simulink model "gm_UZ_EnDat"  (R2023b)
settings: Solver=FixedStepDiscrete  StartTime=0  StopTime=0.002  RelTol=1e-3
model workspace (MAT data in the model file):
  Select = 0
libraries: hdlsllib x314, hdlmdlgenlib x10, simulink x7, simulink_extras x3
(part 6 of 7)

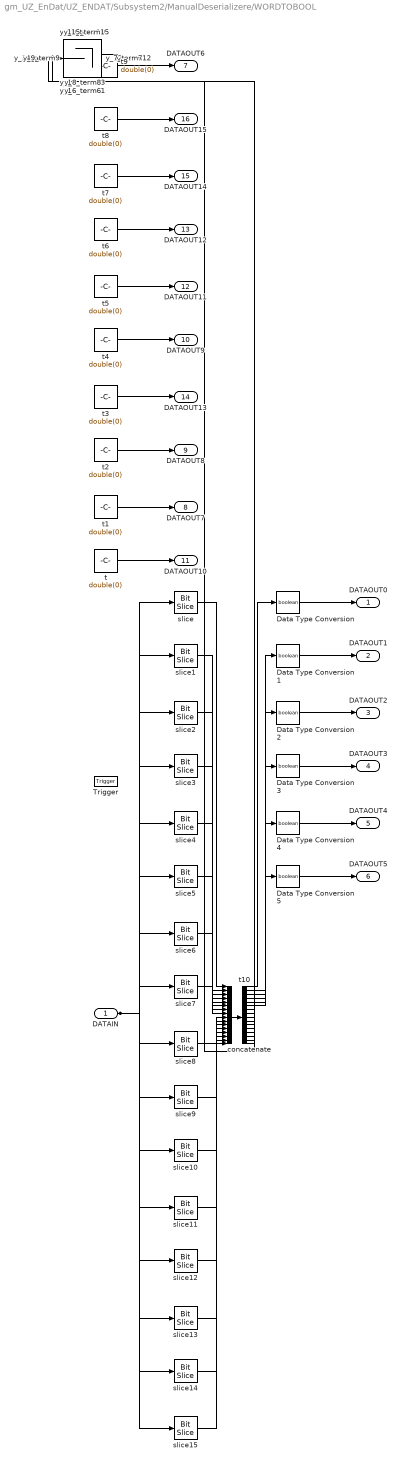
== system gm_UZ_EnDat/UZ_ENDAT/Subsystem2/ManualDeserializere/WORDTOBOOL ==
  DATAIN : Inport  OutDataTypeStr=uint16  PortDimensions=1
  Trigger : TriggerPort  TriggerType=falling  VariantControl=(inherit)  OutputDataType=int8  InitialTriggerSignalState=positive  PortDimensions=1  OutDataTypeStr=boolean
  Data Type Conversion{,1..5} (6 alike) : DataTypeConversion  OutDataTypeStr=boolean  SaturateOnIntegerOverflow=off  RndMeth=Floor
  concatenate : Concatenate  NumInputs=16  Mode=Multidimensional array  ConcatenateDimension=2
  slice : hdlsllib/Logic and Bit Operations/Bit Slice  lidx=double(0)  ridx=double(0)
  slice1 : hdlsllib/Logic and Bit Operations/Bit Slice  lidx=double(1)  ridx=double(1)
  slice10 : hdlsllib/Logic and Bit Operations/Bit Slice  lidx=double(10)  ridx=double(10)
  slice11 : hdlsllib/Logic and Bit Operations/Bit Slice  lidx=double(11)  ridx=double(11)
  slice12 : hdlsllib/Logic and Bit Operations/Bit Slice  lidx=double(12)  ridx=double(12)
  slice13 : hdlsllib/Logic and Bit Operations/Bit Slice  lidx=double(13)  ridx=double(13)
  slice14 : hdlsllib/Logic and Bit Operations/Bit Slice  lidx=double(14)  ridx=double(14)
  slice15 : hdlsllib/Logic and Bit Operations/Bit Slice  lidx=double(15)  ridx=double(15)
  slice2 : hdlsllib/Logic and Bit Operations/Bit Slice  lidx=double(2)  ridx=double(2)
  slice3 : hdlsllib/Logic and Bit Operations/Bit Slice  lidx=double(3)  ridx=double(3)
  slice4 : hdlsllib/Logic and Bit Operations/Bit Slice  lidx=double(4)  ridx=double(4)
  slice5 : hdlsllib/Logic and Bit Operations/Bit Slice  lidx=double(5)  ridx=double(5)
  slice6 : hdlsllib/Logic and Bit Operations/Bit Slice  lidx=double(6)  ridx=double(6)
  slice7 : hdlsllib/Logic and Bit Operations/Bit Slice  lidx=double(7)  ridx=double(7)
  slice8 : hdlsllib/Logic and Bit Operations/Bit Slice  lidx=double(8)  ridx=double(8)
  slice9 : hdlsllib/Logic and Bit Operations/Bit Slice  lidx=double(9)  ridx=double(9)
  t{,1..9} (10 alike) : Constant  Value=double(0)  OutDataTypeStr=boolean  SampleTime=-1
  t10 : Demux  Outputs=16
  y_10_term10 : Terminator
  y_11_term11 : Terminator
  y_12_term12 : Terminator
  y_13_term13 : Terminator
  y_14_term14 : Terminator
  y_15_term15 : Terminator
  y_6_term6 : Terminator
  y_7_term7 : Terminator
  y_8_term8 : Terminator
  y_9_term9 : Terminator
  DATAOUT0 : Outport  InitialOutput=0
  DATAOUT1 : Outport  Port=2  InitialOutput=0
  DATAOUT2 : Outport  Port=3  InitialOutput=0
  DATAOUT3 : Outport  Port=4  InitialOutput=0
  DATAOUT4 : Outport  Port=5  InitialOutput=0
  DATAOUT5 : Outport  Port=6  InitialOutput=0
  DATAOUT6 : Outport  Port=7  InitialOutput=0
  DATAOUT7 : Outport  Port=8  InitialOutput=0
  DATAOUT8 : Outport  Port=9  InitialOutput=0
  DATAOUT9 : Outport  Port=10  InitialOutput=0
  DATAOUT10 : Outport  Port=11  InitialOutput=0
  DATAOUT11 : Outport  Port=12  InitialOutput=0
  DATAOUT12 : Outport  Port=13  InitialOutput=0
  DATAOUT13 : Outport  Port=14  InitialOutput=0
  DATAOUT14 : Outport  Port=15  InitialOutput=0
  DATAOUT15 : Outport  Port=16  InitialOutput=0
  wires:
  DATAIN/1 -> slice15/1, slice14/1, slice13/1, slice12/1, slice11/1, slice10/1, slice9/1, slice8/1, slice7/1, slice6/1, slice5/1, slice4/1, slice3/1, slice2/1, slice1/1, slice/1
  Data Type Conversion/1 -> DATAOUT0/1
  Data Type Conversion1/1 -> DATAOUT1/1
  t/1 -> DATAOUT10/1
  t5/1 -> DATAOUT11/1
  t6/1 -> DATAOUT12/1
  t3/1 -> DATAOUT13/1
  t7/1 -> DATAOUT14/1
  t8/1 -> DATAOUT15/1
  Data Type Conversion2/1 -> DATAOUT2/1
  Data Type Conversion3/1 -> DATAOUT3/1
  Data Type Conversion4/1 -> DATAOUT4/1
  Data Type Conversion5/1 -> DATAOUT5/1
  t9/1 -> DATAOUT6/1
  t1/1 -> DATAOUT7/1
  t2/1 -> DATAOUT8/1
  t4/1 -> DATAOUT9/1
  concatenate/1 -> t10/1
  t10/1 -> Data Type Conversion/1
  t10/2 -> Data Type Conversion1/1
  t10/3 -> Data Type Conversion2/1
  t10/4 -> Data Type Conversion3/1
  t10/5 -> Data Type Conversion4/1
  t10/6 -> Data Type Conversion5/1
  t10/7 -> y_6_term6/1
  t10/8 -> y_7_term7/1
  t10/9 -> y_8_term8/1
  t10/10 -> y_9_term9/1
  t10/11 -> y_10_term10/1
  t10/12 -> y_11_term11/1
  t10/13 -> y_12_term12/1
  t10/14 -> y_13_term13/1
  t10/15 -> y_14_term14/1
  t10/16 -> y_15_term15/1
  slice/1 -> concatenate/1
  slice1/1 -> concatenate/2
  slice2/1 -> concatenate/3
  slice3/1 -> concatenate/4
  slice4/1 -> concatenate/5
  slice5/1 -> concatenate/6
  slice6/1 -> concatenate/7
  slice7/1 -> concatenate/8
  slice8/1 -> concatenate/9
  slice9/1 -> concatenate/10
  slice10/1 -> concatenate/11
  slice11/1 -> concatenate/12
  slice12/1 -> concatenate/13
  slice13/1 -> concatenate/14
  slice14/1 -> concatenate/15
  slice15/1 -> concatenate/16

== system gm_UZ_EnDat/UZ_ENDAT/Subsystem2/ManualDeserializere/ramwatcher ==
  In1 : Inport  OutMin=0  OutMax=32000  OutDataTypeStr=uint16  PortDimensions=1  LockScale=on
  reset : Inport  Port=2  OutMin=0  OutMax=1  OutDataTypeStr=boolean  PortDimensions=1  LockScale=on
  Trigger : TriggerPort  VariantControl=(inherit)  OutputDataType=int8  InitialTriggerSignalState=zero  PortDimensions=1  OutDataTypeStr=boolean
  Constant2 : Constant  Value=0  OutDataTypeStr=uint16  SampleTime=-1
  Increment Stored Integer : Subsystem  mask(Stored Integer Value Increment){}
      mask help: Simulink:masks:StoredIntegerValueIncrement_MD
      mask Display: disp('Q++')
  Index Vector1 : MultiPortSwitch  DataPortOrder=Zero-based contiguous  Inputs=2  DiagnosticForDefault=None  zeroidx=on  OutDataTypeStr=uint16  SaturateOnIntegerOverflow=off  InputSameDT=off
  SEL : Outport  InitialOutput=0
  wires:
  In1/1 -> Increment Stored Integer/1(u)
  reset/1 -> Index Vector1/1
  Constant2/1 -> Index Vector1/3
  Increment Stored Integer/1(y) -> Index Vector1/2
  Index Vector1/1 -> SEL/1

== system gm_UZ_EnDat/UZ_ENDAT/timingprovider/CLKCNTER_POSCNTR/Positional_Counter ==
  valueout : Inport  OutDataTypeStr=uint32  PortDimensions=1
  Trigger : TriggerPort  VariantControl=(inherit)  InitialTriggerSignalState=zero  PortDimensions=1  OutDataTypeStr=boolean
  Increment Stored Integer : Subsystem  mask(Stored Integer Value Increment){}
      mask help: Simulink:masks:StoredIntegerValueIncrement_MD
      mask Display: disp('Q++')
  divider : Outport  InitialOutput=0
  wires:
  valueout/1 -> Increment Stored Integer/1(u)
  Increment Stored Integer/1(y) -> divider/1

== system gm_UZ_EnDat/UZ_ENDAT/timingprovider/CLKCNTER_POSCNTR/SetZero32modified ==
  valin : Inport  OutDataTypeStr=uint32  PortDimensions=1
  setzero : Inport  Port=2  OutDataTypeStr=boolean  PortDimensions=1
  Trigger : TriggerPort  TriggerType=either  VariantControl=(inherit)  PortDimensions=1  OutDataTypeStr=boolean
  Constant2 : Constant  Value=0  OutDataTypeStr=uint32  SampleTime=-1
  Index Vector1 : MultiPortSwitch  DataPortOrder=Zero-based contiguous  Inputs=2  DiagnosticForDefault=None  zeroidx=on  OutDataTypeStr=uint32  SaturateOnIntegerOverflow=off  InputSameDT=off
  valueout : Outport  InitialOutput=0  VectorParamsAs1DForOutWhenUnconnected=off
  wires:
  valin/1 -> Index Vector1/2
  setzero/1 -> Index Vector1/1
  Constant2/1 -> Index Vector1/3
  Index Vector1/1 -> valueout/1

== system gm_UZ_EnDat/UZ_ENDAT/timingprovider/CLKCNTER_POSCNTR/SetZero32modified1 ==
  valin : Inport  OutDataTypeStr=uint32  PortDimensions=1
  setzero : Inport  Port=2  OutDataTypeStr=boolean  PortDimensions=1
  Trigger : TriggerPort  TriggerType=either  VariantControl=(inherit)  PortDimensions=1  OutDataTypeStr=boolean
  Constant2 : Constant  Value=0  OutDataTypeStr=uint32  SampleTime=-1
  Index Vector1 : MultiPortSwitch  DataPortOrder=Zero-based contiguous  Inputs=2  DiagnosticForDefault=None  zeroidx=on  OutDataTypeStr=uint32  SaturateOnIntegerOverflow=off  InputSameDT=off
  valueout : Outport  InitialOutput=0  VectorParamsAs1DForOutWhenUnconnected=off
  wires:
  valin/1 -> Index Vector1/2
  setzero/1 -> Index Vector1/1
  Constant2/1 -> Index Vector1/3
  Index Vector1/1 -> valueout/1

== system gm_UZ_EnDat/UZ_ENDAT/timingprovider/CLKCNTER_POSCNTR1/Positional_Counter ==
  valueout : Inport  OutDataTypeStr=uint32  PortDimensions=1
  Trigger : TriggerPort  VariantControl=(inherit)  InitialTriggerSignalState=zero  PortDimensions=1  OutDataTypeStr=boolean
  Increment Stored Integer : Subsystem  mask(Stored Integer Value Increment){}
      mask help: Simulink:masks:StoredIntegerValueIncrement_MD
      mask Display: disp('Q++')
  divider : Outport  InitialOutput=0
  wires:
  Increment Stored Integer/1(y) -> divider/1
  valueout/1 -> Increment Stored Integer/1(u)

== system gm_UZ_EnDat/UZ_ENDAT/timingprovider/CLKCNTER_POSCNTR1/SetZero32modified ==
  valin : Inport  OutDataTypeStr=uint32  PortDimensions=1
  setzero : Inport  Port=2  OutDataTypeStr=boolean  PortDimensions=1
  Trigger : TriggerPort  TriggerType=either  VariantControl=(inherit)  PortDimensions=1  OutDataTypeStr=boolean
  Constant2 : Constant  Value=0  OutDataTypeStr=uint32  SampleTime=-1
  Index Vector1 : MultiPortSwitch  DataPortOrder=Zero-based contiguous  Inputs=2  DiagnosticForDefault=None  zeroidx=on  OutDataTypeStr=uint32  SaturateOnIntegerOverflow=off  InputSameDT=off
  valueout : Outport  InitialOutput=0  VectorParamsAs1DForOutWhenUnconnected=off
  wires:
  Constant2/1 -> Index Vector1/3
  Index Vector1/1 -> valueout/1
  valin/1 -> Index Vector1/2
  setzero/1 -> Index Vector1/1

== system gm_UZ_EnDat/UZ_ENDAT/timingprovider/Subsystem2/Compare To Constant1 ==
  u : Inport  OutDataTypeStr=uint32  SampleTime=1e-08
  Compare : RelationalOperator  Operator===  OutDataTypeStr=boolean
  Constant : Constant  DisableCoverage=on  Value=const  OutDataTypeStr=Inherit: Inherit via back propagation  SampleTime=-1
  y : Outport  SampleTime=1e-08
  wires:
  u/1 -> Compare/1
  Compare/1 -> y/1
  Constant/1 -> Compare/2

== system gm_UZ_EnDat/UZ_ENDAT/timingprovider/Subsystem2/Detect Increase ==
  note: U(k)
  note: Edge
  U : Inport  OutDataTypeStr=boolean  SampleTime=1e-08
  Delay Input1 : UnitDelay  SampleTime=1e-08
  FixPt Relational Operator : RelationalOperator  Operator=>  OutDataTypeStr=boolean  SampleTime=1e-08  InputSameDT=off
  Y : Outport  SampleTime=1e-08
  wires:
  U/1 -> FixPt Relational Operator/1, Delay Input1/1
  Delay Input1/1 -> FixPt Relational Operator/2
  FixPt Relational Operator/1 -> Y/1

== system gm_UZ_EnDat/UZ_ENDAT/timingprovider/Subsystem3/Compare To Constant1 ==
  u : Inport  OutDataTypeStr=uint32  SampleTime=1e-08
  Compare : RelationalOperator  Operator===  OutDataTypeStr=boolean
  Constant : Constant  DisableCoverage=on  Value=const  OutDataTypeStr=Inherit: Inherit via back propagation  SampleTime=-1
  y : Outport  SampleTime=1e-08
  wires:
  u/1 -> Compare/1
  Compare/1 -> y/1
  Constant/1 -> Compare/2

== system gm_UZ_EnDat/UZ_ENDAT/timingprovider/Subsystem3/Detect Increase ==
  note: U(k)
  note: Edge
  U : Inport  OutDataTypeStr=boolean  SampleTime=1e-08
  Delay Input1 : UnitDelay  SampleTime=1e-08
  FixPt Relational Operator : RelationalOperator  Operator=>  OutDataTypeStr=boolean  SampleTime=1e-08  InputSameDT=off
  Y : Outport  SampleTime=1e-08
  wires:
  U/1 -> FixPt Relational Operator/1, Delay Input1/1
  Delay Input1/1 -> FixPt Relational Operator/2
  FixPt Relational Operator/1 -> Y/1

== system gm_UZ_EnDat/UZ_ENDAT/3timestorage/Triggered Subsystem/Counter Limited/Increment Real World ==
  u : Inport  OutDataTypeStr=uint8
  FixPt Constant : Constant  OutDataTypeStr=uint8  SampleTime=-1
  FixPt Data Type Duplicate : DataTypeDuplicate  DisableCoverage=on  NumInputPorts=3
  FixPt Sum1 : Sum  OutDataTypeStr=uint8  AccumDataTypeStr=uint8
  y : Outport  InitialOutput=0
  wires:
  u/1 -> FixPt Sum1/1, FixPt Data Type Duplicate/2
  FixPt Constant/1 -> FixPt Sum1/2, FixPt Data Type Duplicate/3
  FixPt Sum1/1 -> FixPt Data Type Duplicate/1, y/1

== system gm_UZ_EnDat/UZ_ENDAT/3timestorage/Triggered Subsystem/Counter Limited/Wrap To Zero ==
  note: U(k)
  U : Inport  OutDataTypeStr=uint8
  Constant : Constant  Value=0  OutDataTypeStr=uint8  SampleTime=-1
  FixPt Data Type Duplicate1 : DataTypeDuplicate  DisableCoverage=on  NumInputPorts=3
  FixPt Switch : Switch  Criteria=u2 > Threshold  Threshold=double(2)  OutDataTypeStr=uint8  SaturateOnIntegerOverflow=off  InputSameDT=off
  Y : Outport  InitialOutput=0
  wires:
  U/1 -> FixPt Switch/3, FixPt Switch/2, FixPt Data Type Duplicate1/2
  Constant/1 -> FixPt Switch/1, FixPt Data Type Duplicate1/3
  FixPt Switch/1 -> FixPt Data Type Duplicate1/1, Y/1

== system gm_UZ_EnDat/UZ_ENDAT/ManualSerialize/padder/nibblepadding1/padding1 ==
  in : Inport  OutDataTypeStr=fixdt(0, 64, 0)  PortDimensions=1  SampleTime=1e-08
  Bit Shift2 : hdlsllib/Logic and Bit Operations/Bit Shift  mode=Shift Right Logical  N=double(1)
  Bit Slice2 : hdlsllib/Logic and Bit Operations/Bit Slice  lidx=double(0)  ridx=double(0)
  Data Type Conversion2 : DataTypeConversion  OutDataTypeStr=boolean  RndMeth=Nearest  SampleTime=1e-08  SaturateOnIntegerOverflow=off
  Switch2 : Switch  Criteria=u2 > Threshold  Threshold=double(0)  OutDataTypeStr=fixdt(0, 64, 0)  SampleTime=1e-08  SaturateOnIntegerOverflow=off  InputSameDT=off
  out : Outport  SampleTime=1e-08
  wires:
  in/1 -> Switch2/1, Bit Slice2/1, Bit Shift2/1
  Bit Shift2/1 -> Switch2/3
  Bit Slice2/1 -> Data Type Conversion2/1
  Data Type Conversion2/1 -> Switch2/2
  Switch2/1 -> out/1

== system gm_UZ_EnDat/UZ_ENDAT/ManualSerialize/padder/nibblepadding1/padding2 ==
  in : Inport  OutDataTypeStr=fixdt(0, 64, 0)  PortDimensions=1  SampleTime=1e-08
  Bit Shift2 : hdlsllib/Logic and Bit Operations/Bit Shift  mode=Shift Right Logical  N=double(1)
  Bit Slice2 : hdlsllib/Logic and Bit Operations/Bit Slice  lidx=double(0)  ridx=double(0)
  Data Type Conversion2 : DataTypeConversion  OutDataTypeStr=boolean  RndMeth=Nearest  SampleTime=1e-08  SaturateOnIntegerOverflow=off
  Switch2 : Switch  Criteria=u2 > Threshold  Threshold=double(0)  OutDataTypeStr=fixdt(0, 64, 0)  SampleTime=1e-08  SaturateOnIntegerOverflow=off  InputSameDT=off
  out : Outport  SampleTime=1e-08
  wires:
  Switch2/1 -> out/1
  Data Type Conversion2/1 -> Switch2/2
  Bit Slice2/1 -> Data Type Conversion2/1
  Bit Shift2/1 -> Switch2/3
  in/1 -> Bit Shift2/1, Bit Slice2/1, Switch2/1

== system gm_UZ_EnDat/UZ_ENDAT/ManualSerialize/padder/nibblepadding1/padding3 ==
  in : Inport  OutDataTypeStr=fixdt(0, 64, 0)  PortDimensions=1  SampleTime=1e-08
  Bit Shift2 : hdlsllib/Logic and Bit Operations/Bit Shift  mode=Shift Right Logical  N=double(1)
  Bit Slice2 : hdlsllib/Logic and Bit Operations/Bit Slice  lidx=double(0)  ridx=double(0)
  Data Type Conversion2 : DataTypeConversion  OutDataTypeStr=boolean  RndMeth=Nearest  SampleTime=1e-08  SaturateOnIntegerOverflow=off
  Switch2 : Switch  Criteria=u2 > Threshold  Threshold=double(0)  OutDataTypeStr=fixdt(0, 64, 0)  SampleTime=1e-08  SaturateOnIntegerOverflow=off  InputSameDT=off
  out : Outport  SampleTime=1e-08
  wires:
  Switch2/1 -> out/1
  Data Type Conversion2/1 -> Switch2/2
  Bit Slice2/1 -> Data Type Conversion2/1
  Bit Shift2/1 -> Switch2/3
  in/1 -> Bit Shift2/1, Bit Slice2/1, Switch2/1

== system gm_UZ_EnDat/UZ_ENDAT/ManualSerialize/padder/nibblepadding10/padding1 ==
  in : Inport  OutDataTypeStr=fixdt(0, 64, 0)  PortDimensions=1  SampleTime=1e-08
  Bit Shift2 : hdlsllib/Logic and Bit Operations/Bit Shift  mode=Shift Right Logical  N=double(1)
  Bit Slice2 : hdlsllib/Logic and Bit Operations/Bit Slice  lidx=double(0)  ridx=double(0)
  Data Type Conversion2 : DataTypeConversion  OutDataTypeStr=boolean  RndMeth=Nearest  SampleTime=1e-08  SaturateOnIntegerOverflow=off
  Switch2 : Switch  Criteria=u2 > Threshold  Threshold=double(0)  OutDataTypeStr=fixdt(0, 64, 0)  SampleTime=1e-08  SaturateOnIntegerOverflow=off  InputSameDT=off
  out : Outport  SampleTime=1e-08
  wires:
  Switch2/1 -> out/1
  Data Type Conversion2/1 -> Switch2/2
  Bit Slice2/1 -> Data Type Conversion2/1
  Bit Shift2/1 -> Switch2/3
  in/1 -> Bit Shift2/1, Bit Slice2/1, Switch2/1

== system gm_UZ_EnDat/UZ_ENDAT/ManualSerialize/padder/nibblepadding10/padding2 ==
  in : Inport  OutDataTypeStr=fixdt(0, 64, 0)  PortDimensions=1  SampleTime=1e-08
  Bit Shift2 : hdlsllib/Logic and Bit Operations/Bit Shift  mode=Shift Right Logical  N=double(1)
  Bit Slice2 : hdlsllib/Logic and Bit Operations/Bit Slice  lidx=double(0)  ridx=double(0)
  Data Type Conversion2 : DataTypeConversion  OutDataTypeStr=boolean  RndMeth=Nearest  SampleTime=1e-08  SaturateOnIntegerOverflow=off
  Switch2 : Switch  Criteria=u2 > Threshold  Threshold=double(0)  OutDataTypeStr=fixdt(0, 64, 0)  SampleTime=1e-08  SaturateOnIntegerOverflow=off  InputSameDT=off
  out : Outport  SampleTime=1e-08
  wires:
  in/1 -> Switch2/1, Bit Slice2/1, Bit Shift2/1
  Bit Shift2/1 -> Switch2/3
  Bit Slice2/1 -> Data Type Conversion2/1
  Data Type Conversion2/1 -> Switch2/2
  Switch2/1 -> out/1

== system gm_UZ_EnDat/UZ_ENDAT/ManualSerialize/padder/nibblepadding10/padding3 ==
  in : Inport  OutDataTypeStr=fixdt(0, 64, 0)  PortDimensions=1  SampleTime=1e-08
  Bit Shift2 : hdlsllib/Logic and Bit Operations/Bit Shift  mode=Shift Right Logical  N=double(1)
  Bit Slice2 : hdlsllib/Logic and Bit Operations/Bit Slice  lidx=double(0)  ridx=double(0)
  Data Type Conversion2 : DataTypeConversion  OutDataTypeStr=boolean  RndMeth=Nearest  SampleTime=1e-08  SaturateOnIntegerOverflow=off
  Switch2 : Switch  Criteria=u2 > Threshold  Threshold=double(0)  OutDataTypeStr=fixdt(0, 64, 0)  SampleTime=1e-08  SaturateOnIntegerOverflow=off  InputSameDT=off
  out : Outport  SampleTime=1e-08
  wires:
  in/1 -> Switch2/1, Bit Slice2/1, Bit Shift2/1
  Bit Shift2/1 -> Switch2/3
  Bit Slice2/1 -> Data Type Conversion2/1
  Data Type Conversion2/1 -> Switch2/2
  Switch2/1 -> out/1

== system gm_UZ_EnDat/UZ_ENDAT/ManualSerialize/padder/nibblepadding11/padding1 ==
  in : Inport  OutDataTypeStr=fixdt(0, 64, 0)  PortDimensions=1  SampleTime=1e-08
  Bit Shift2 : hdlsllib/Logic and Bit Operations/Bit Shift  mode=Shift Right Logical  N=double(1)
  Bit Slice2 : hdlsllib/Logic and Bit Operations/Bit Slice  lidx=double(0)  ridx=double(0)
  Data Type Conversion2 : DataTypeConversion  OutDataTypeStr=boolean  RndMeth=Nearest  SampleTime=1e-08  SaturateOnIntegerOverflow=off
  Switch2 : Switch  Criteria=u2 > Threshold  Threshold=double(0)  OutDataTypeStr=fixdt(0, 64, 0)  SampleTime=1e-08  SaturateOnIntegerOverflow=off  InputSameDT=off
  out : Outport  SampleTime=1e-08
  wires:
  Switch2/1 -> out/1
  Data Type Conversion2/1 -> Switch2/2
  Bit Slice2/1 -> Data Type Conversion2/1
  Bit Shift2/1 -> Switch2/3
  in/1 -> Bit Shift2/1, Bit Slice2/1, Switch2/1

== system gm_UZ_EnDat/UZ_ENDAT/ManualSerialize/padder/nibblepadding11/padding2 ==
  in : Inport  OutDataTypeStr=fixdt(0, 64, 0)  PortDimensions=1  SampleTime=1e-08
  Bit Shift2 : hdlsllib/Logic and Bit Operations/Bit Shift  mode=Shift Right Logical  N=double(1)
  Bit Slice2 : hdlsllib/Logic and Bit Operations/Bit Slice  lidx=double(0)  ridx=double(0)
  Data Type Conversion2 : DataTypeConversion  OutDataTypeStr=boolean  RndMeth=Nearest  SampleTime=1e-08  SaturateOnIntegerOverflow=off
  Switch2 : Switch  Criteria=u2 > Threshold  Threshold=double(0)  OutDataTypeStr=fixdt(0, 64, 0)  SampleTime=1e-08  SaturateOnIntegerOverflow=off  InputSameDT=off
  out : Outport  SampleTime=1e-08
  wires:
  in/1 -> Switch2/1, Bit Slice2/1, Bit Shift2/1
  Bit Shift2/1 -> Switch2/3
  Bit Slice2/1 -> Data Type Conversion2/1
  Data Type Conversion2/1 -> Switch2/2
  Switch2/1 -> out/1

== system gm_UZ_EnDat/UZ_ENDAT/ManualSerialize/padder/nibblepadding11/padding3 ==
  in : Inport  OutDataTypeStr=fixdt(0, 64, 0)  PortDimensions=1  SampleTime=1e-08
  Bit Shift2 : hdlsllib/Logic and Bit Operations/Bit Shift  mode=Shift Right Logical  N=double(1)
  Bit Slice2 : hdlsllib/Logic and Bit Operations/Bit Slice  lidx=double(0)  ridx=double(0)
  Data Type Conversion2 : DataTypeConversion  OutDataTypeStr=boolean  RndMeth=Nearest  SampleTime=1e-08  SaturateOnIntegerOverflow=off
  Switch2 : Switch  Criteria=u2 > Threshold  Threshold=double(0)  OutDataTypeStr=fixdt(0, 64, 0)  SampleTime=1e-08  SaturateOnIntegerOverflow=off  InputSameDT=off
  out : Outport  SampleTime=1e-08
  wires:
  in/1 -> Switch2/1, Bit Slice2/1, Bit Shift2/1
  Bit Shift2/1 -> Switch2/3
  Bit Slice2/1 -> Data Type Conversion2/1
  Data Type Conversion2/1 -> Switch2/2
  Switch2/1 -> out/1

== system gm_UZ_EnDat/UZ_ENDAT/ManualSerialize/padder/nibblepadding12/padding1 ==
  in : Inport  OutDataTypeStr=fixdt(0, 64, 0)  PortDimensions=1  SampleTime=1e-08
  Bit Shift2 : hdlsllib/Logic and Bit Operations/Bit Shift  mode=Shift Right Logical  N=double(1)
  Bit Slice2 : hdlsllib/Logic and Bit Operations/Bit Slice  lidx=double(0)  ridx=double(0)
  Data Type Conversion2 : DataTypeConversion  OutDataTypeStr=boolean  RndMeth=Nearest  SampleTime=1e-08  SaturateOnIntegerOverflow=off
  Switch2 : Switch  Criteria=u2 > Threshold  Threshold=double(0)  OutDataTypeStr=fixdt(0, 64, 0)  SampleTime=1e-08  SaturateOnIntegerOverflow=off  InputSameDT=off
  out : Outport  SampleTime=1e-08
  wires:
  Switch2/1 -> out/1
  Data Type Conversion2/1 -> Switch2/2
  Bit Slice2/1 -> Data Type Conversion2/1
  Bit Shift2/1 -> Switch2/3
  in/1 -> Bit Shift2/1, Bit Slice2/1, Switch2/1

== system gm_UZ_EnDat/UZ_ENDAT/ManualSerialize/padder/nibblepadding12/padding2 ==
  in : Inport  OutDataTypeStr=fixdt(0, 64, 0)  PortDimensions=1  SampleTime=1e-08
  Bit Shift2 : hdlsllib/Logic and Bit Operations/Bit Shift  mode=Shift Right Logical  N=double(1)
  Bit Slice2 : hdlsllib/Logic and Bit Operations/Bit Slice  lidx=double(0)  ridx=double(0)
  Data Type Conversion2 : DataTypeConversion  OutDataTypeStr=boolean  RndMeth=Nearest  SampleTime=1e-08  SaturateOnIntegerOverflow=off
  Switch2 : Switch  Criteria=u2 > Threshold  Threshold=double(0)  OutDataTypeStr=fixdt(0, 64, 0)  SampleTime=1e-08  SaturateOnIntegerOverflow=off  InputSameDT=off
  out : Outport  SampleTime=1e-08
  wires:
  in/1 -> Switch2/1, Bit Slice2/1, Bit Shift2/1
  Bit Shift2/1 -> Switch2/3
  Bit Slice2/1 -> Data Type Conversion2/1
  Data Type Conversion2/1 -> Switch2/2
  Switch2/1 -> out/1

== system gm_UZ_EnDat/UZ_ENDAT/ManualSerialize/padder/nibblepadding12/padding3 ==
  in : Inport  OutDataTypeStr=fixdt(0, 64, 0)  PortDimensions=1  SampleTime=1e-08
  Bit Shift2 : hdlsllib/Logic and Bit Operations/Bit Shift  mode=Shift Right Logical  N=double(1)
  Bit Slice2 : hdlsllib/Logic and Bit Operations/Bit Slice  lidx=double(0)  ridx=double(0)
  Data Type Conversion2 : DataTypeConversion  OutDataTypeStr=boolean  RndMeth=Nearest  SampleTime=1e-08  SaturateOnIntegerOverflow=off
  Switch2 : Switch  Criteria=u2 > Threshold  Threshold=double(0)  OutDataTypeStr=fixdt(0, 64, 0)  SampleTime=1e-08  SaturateOnIntegerOverflow=off  InputSameDT=off
  out : Outport  SampleTime=1e-08
  wires:
  in/1 -> Switch2/1, Bit Slice2/1, Bit Shift2/1
  Bit Shift2/1 -> Switch2/3
  Bit Slice2/1 -> Data Type Conversion2/1
  Data Type Conversion2/1 -> Switch2/2
  Switch2/1 -> out/1

== system gm_UZ_EnDat/UZ_ENDAT/ManualSerialize/padder/nibblepadding13/padding1 ==
  in : Inport  OutDataTypeStr=fixdt(0, 64, 0)  PortDimensions=1  SampleTime=1e-08
  Bit Shift2 : hdlsllib/Logic and Bit Operations/Bit Shift  mode=Shift Right Logical  N=double(1)
  Bit Slice2 : hdlsllib/Logic and Bit Operations/Bit Slice  lidx=double(0)  ridx=double(0)
  Data Type Conversion2 : DataTypeConversion  OutDataTypeStr=boolean  RndMeth=Nearest  SampleTime=1e-08  SaturateOnIntegerOverflow=off
  Switch2 : Switch  Criteria=u2 > Threshold  Threshold=double(0)  OutDataTypeStr=fixdt(0, 64, 0)  SampleTime=1e-08  SaturateOnIntegerOverflow=off  InputSameDT=off
  out : Outport  SampleTime=1e-08
  wires:
  Switch2/1 -> out/1
  Data Type Conversion2/1 -> Switch2/2
  Bit Slice2/1 -> Data Type Conversion2/1
  Bit Shift2/1 -> Switch2/3
  in/1 -> Bit Shift2/1, Bit Slice2/1, Switch2/1

== system gm_UZ_EnDat/UZ_ENDAT/ManualSerialize/padder/nibblepadding13/padding2 ==
  in : Inport  OutDataTypeStr=fixdt(0, 64, 0)  PortDimensions=1  SampleTime=1e-08
  Bit Shift2 : hdlsllib/Logic and Bit Operations/Bit Shift  mode=Shift Right Logical  N=double(1)
  Bit Slice2 : hdlsllib/Logic and Bit Operations/Bit Slice  lidx=double(0)  ridx=double(0)
  Data Type Conversion2 : DataTypeConversion  OutDataTypeStr=boolean  RndMeth=Nearest  SampleTime=1e-08  SaturateOnIntegerOverflow=off
  Switch2 : Switch  Criteria=u2 > Threshold  Threshold=double(0)  OutDataTypeStr=fixdt(0, 64, 0)  SampleTime=1e-08  SaturateOnIntegerOverflow=off  InputSameDT=off
  out : Outport  SampleTime=1e-08
  wires:
  in/1 -> Switch2/1, Bit Slice2/1, Bit Shift2/1
  Bit Shift2/1 -> Switch2/3
  Bit Slice2/1 -> Data Type Conversion2/1
  Data Type Conversion2/1 -> Switch2/2
  Switch2/1 -> out/1

== system gm_UZ_EnDat/UZ_ENDAT/ManualSerialize/padder/nibblepadding13/padding3 ==
  in : Inport  OutDataTypeStr=fixdt(0, 64, 0)  PortDimensions=1  SampleTime=1e-08
  Bit Shift2 : hdlsllib/Logic and Bit Operations/Bit Shift  mode=Shift Right Logical  N=double(1)
  Bit Slice2 : hdlsllib/Logic and Bit Operations/Bit Slice  lidx=double(0)  ridx=double(0)
  Data Type Conversion2 : DataTypeConversion  OutDataTypeStr=boolean  RndMeth=Nearest  SampleTime=1e-08  SaturateOnIntegerOverflow=off
  Switch2 : Switch  Criteria=u2 > Threshold  Threshold=double(0)  OutDataTypeStr=fixdt(0, 64, 0)  SampleTime=1e-08  SaturateOnIntegerOverflow=off  InputSameDT=off
  out : Outport  SampleTime=1e-08
  wires:
  in/1 -> Switch2/1, Bit Slice2/1, Bit Shift2/1
  Bit Shift2/1 -> Switch2/3
  Bit Slice2/1 -> Data Type Conversion2/1
  Data Type Conversion2/1 -> Switch2/2
  Switch2/1 -> out/1

== system gm_UZ_EnDat/UZ_ENDAT/ManualSerialize/padder/nibblepadding14/padding1 ==
  in : Inport  OutDataTypeStr=fixdt(0, 64, 0)  PortDimensions=1  SampleTime=1e-08
  Bit Shift2 : hdlsllib/Logic and Bit Operations/Bit Shift  mode=Shift Right Logical  N=double(1)
  Bit Slice2 : hdlsllib/Logic and Bit Operations/Bit Slice  lidx=double(0)  ridx=double(0)
  Data Type Conversion2 : DataTypeConversion  OutDataTypeStr=boolean  RndMeth=Nearest  SampleTime=1e-08  SaturateOnIntegerOverflow=off
  Switch2 : Switch  Criteria=u2 > Threshold  Threshold=double(0)  OutDataTypeStr=fixdt(0, 64, 0)  SampleTime=1e-08  SaturateOnIntegerOverflow=off  InputSameDT=off
  out : Outport  SampleTime=1e-08
  wires:
  Switch2/1 -> out/1
  Data Type Conversion2/1 -> Switch2/2
  Bit Slice2/1 -> Data Type Conversion2/1
  Bit Shift2/1 -> Switch2/3
  in/1 -> Bit Shift2/1, Bit Slice2/1, Switch2/1

== system gm_UZ_EnDat/UZ_ENDAT/ManualSerialize/padder/nibblepadding14/padding2 ==
  in : Inport  OutDataTypeStr=fixdt(0, 64, 0)  PortDimensions=1  SampleTime=1e-08
  Bit Shift2 : hdlsllib/Logic and Bit Operations/Bit Shift  mode=Shift Right Logical  N=double(1)
  Bit Slice2 : hdlsllib/Logic and Bit Operations/Bit Slice  lidx=double(0)  ridx=double(0)
  Data Type Conversion2 : DataTypeConversion  OutDataTypeStr=boolean  RndMeth=Nearest  SampleTime=1e-08  SaturateOnIntegerOverflow=off
  Switch2 : Switch  Criteria=u2 > Threshold  Threshold=double(0)  OutDataTypeStr=fixdt(0, 64, 0)  SampleTime=1e-08  SaturateOnIntegerOverflow=off  InputSameDT=off
  out : Outport  SampleTime=1e-08
  wires:
  in/1 -> Switch2/1, Bit Slice2/1, Bit Shift2/1
  Bit Shift2/1 -> Switch2/3
  Bit Slice2/1 -> Data Type Conversion2/1
  Data Type Conversion2/1 -> Switch2/2
  Switch2/1 -> out/1

== system gm_UZ_EnDat/UZ_ENDAT/ManualSerialize/padder/nibblepadding14/padding3 ==
  in : Inport  OutDataTypeStr=fixdt(0, 64, 0)  PortDimensions=1  SampleTime=1e-08
  Bit Shift2 : hdlsllib/Logic and Bit Operations/Bit Shift  mode=Shift Right Logical  N=double(1)
  Bit Slice2 : hdlsllib/Logic and Bit Operations/Bit Slice  lidx=double(0)  ridx=double(0)
  Data Type Conversion2 : DataTypeConversion  OutDataTypeStr=boolean  RndMeth=Nearest  SampleTime=1e-08  SaturateOnIntegerOverflow=off
  Switch2 : Switch  Criteria=u2 > Threshold  Threshold=double(0)  OutDataTypeStr=fixdt(0, 64, 0)  SampleTime=1e-08  SaturateOnIntegerOverflow=off  InputSameDT=off
  out : Outport  SampleTime=1e-08
  wires:
  in/1 -> Switch2/1, Bit Slice2/1, Bit Shift2/1
  Bit Shift2/1 -> Switch2/3
  Bit Slice2/1 -> Data Type Conversion2/1
  Data Type Conversion2/1 -> Switch2/2
  Switch2/1 -> out/1

== system gm_UZ_EnDat/UZ_ENDAT/ManualSerialize/padder/nibblepadding15/padding1 ==
  in : Inport  OutDataTypeStr=fixdt(0, 64, 0)  PortDimensions=1  SampleTime=1e-08
  Bit Shift2 : hdlsllib/Logic and Bit Operations/Bit Shift  mode=Shift Right Logical  N=double(1)
  Bit Slice2 : hdlsllib/Logic and Bit Operations/Bit Slice  lidx=double(0)  ridx=double(0)
  Data Type Conversion2 : DataTypeConversion  OutDataTypeStr=boolean  RndMeth=Nearest  SampleTime=1e-08  SaturateOnIntegerOverflow=off
  Switch2 : Switch  Criteria=u2 > Threshold  Threshold=double(0)  OutDataTypeStr=fixdt(0, 64, 0)  SampleTime=1e-08  SaturateOnIntegerOverflow=off  InputSameDT=off
  out : Outport  SampleTime=1e-08
  wires:
  Switch2/1 -> out/1
  Data Type Conversion2/1 -> Switch2/2
  Bit Slice2/1 -> Data Type Conversion2/1
  Bit Shift2/1 -> Switch2/3
  in/1 -> Bit Shift2/1, Bit Slice2/1, Switch2/1

== system gm_UZ_EnDat/UZ_ENDAT/ManualSerialize/padder/nibblepadding15/padding2 ==
  in : Inport  OutDataTypeStr=fixdt(0, 64, 0)  PortDimensions=1  SampleTime=1e-08
  Bit Shift2 : hdlsllib/Logic and Bit Operations/Bit Shift  mode=Shift Right Logical  N=double(1)
  Bit Slice2 : hdlsllib/Logic and Bit Operations/Bit Slice  lidx=double(0)  ridx=double(0)
  Data Type Conversion2 : DataTypeConversion  OutDataTypeStr=boolean  RndMeth=Nearest  SampleTime=1e-08  SaturateOnIntegerOverflow=off
  Switch2 : Switch  Criteria=u2 > Threshold  Threshold=double(0)  OutDataTypeStr=fixdt(0, 64, 0)  SampleTime=1e-08  SaturateOnIntegerOverflow=off  InputSameDT=off
  out : Outport  SampleTime=1e-08
  wires:
  in/1 -> Switch2/1, Bit Slice2/1, Bit Shift2/1
  Bit Shift2/1 -> Switch2/3
  Bit Slice2/1 -> Data Type Conversion2/1
  Data Type Conversion2/1 -> Switch2/2
  Switch2/1 -> out/1

== system gm_UZ_EnDat/UZ_ENDAT/ManualSerialize/padder/nibblepadding15/padding3 ==
  in : Inport  OutDataTypeStr=fixdt(0, 64, 0)  PortDimensions=1  SampleTime=1e-08
  Bit Shift2 : hdlsllib/Logic and Bit Operations/Bit Shift  mode=Shift Right Logical  N=double(1)
  Bit Slice2 : hdlsllib/Logic and Bit Operations/Bit Slice  lidx=double(0)  ridx=double(0)
  Data Type Conversion2 : DataTypeConversion  OutDataTypeStr=boolean  RndMeth=Nearest  SampleTime=1e-08  SaturateOnIntegerOverflow=off
  Switch2 : Switch  Criteria=u2 > Threshold  Threshold=double(0)  OutDataTypeStr=fixdt(0, 64, 0)  SampleTime=1e-08  SaturateOnIntegerOverflow=off  InputSameDT=off
  out : Outport  SampleTime=1e-08
  wires:
  in/1 -> Switch2/1, Bit Slice2/1, Bit Shift2/1
  Bit Shift2/1 -> Switch2/3
  Bit Slice2/1 -> Data Type Conversion2/1
  Data Type Conversion2/1 -> Switch2/2
  Switch2/1 -> out/1

== system gm_UZ_EnDat/UZ_ENDAT/ManualSerialize/padder/nibblepadding16/padding1 ==
  in : Inport  OutDataTypeStr=fixdt(0, 64, 0)  PortDimensions=1  SampleTime=1e-08
  Bit Shift2 : hdlsllib/Logic and Bit Operations/Bit Shift  mode=Shift Right Logical  N=double(1)
  Bit Slice2 : hdlsllib/Logic and Bit Operations/Bit Slice  lidx=double(0)  ridx=double(0)
  Data Type Conversion2 : DataTypeConversion  OutDataTypeStr=boolean  RndMeth=Nearest  SampleTime=1e-08  SaturateOnIntegerOverflow=off
  Switch2 : Switch  Criteria=u2 > Threshold  Threshold=double(0)  OutDataTypeStr=fixdt(0, 64, 0)  SampleTime=1e-08  SaturateOnIntegerOverflow=off  InputSameDT=off
  out : Outport  SampleTime=1e-08
  wires:
  Switch2/1 -> out/1
  Data Type Conversion2/1 -> Switch2/2
  Bit Slice2/1 -> Data Type Conversion2/1
  Bit Shift2/1 -> Switch2/3
  in/1 -> Bit Shift2/1, Bit Slice2/1, Switch2/1

== system gm_UZ_EnDat/UZ_ENDAT/ManualSerialize/padder/nibblepadding16/padding2 ==
  in : Inport  OutDataTypeStr=fixdt(0, 64, 0)  PortDimensions=1  SampleTime=1e-08
  Bit Shift2 : hdlsllib/Logic and Bit Operations/Bit Shift  mode=Shift Right Logical  N=double(1)
  Bit Slice2 : hdlsllib/Logic and Bit Operations/Bit Slice  lidx=double(0)  ridx=double(0)
  Data Type Conversion2 : DataTypeConversion  OutDataTypeStr=boolean  RndMeth=Nearest  SampleTime=1e-08  SaturateOnIntegerOverflow=off
  Switch2 : Switch  Criteria=u2 > Threshold  Threshold=double(0)  OutDataTypeStr=fixdt(0, 64, 0)  SampleTime=1e-08  SaturateOnIntegerOverflow=off  InputSameDT=off
  out : Outport  SampleTime=1e-08
  wires:
  in/1 -> Switch2/1, Bit Slice2/1, Bit Shift2/1
  Bit Shift2/1 -> Switch2/3
  Bit Slice2/1 -> Data Type Conversion2/1
  Data Type Conversion2/1 -> Switch2/2
  Switch2/1 -> out/1

== system gm_UZ_EnDat/UZ_ENDAT/ManualSerialize/padder/nibblepadding16/padding3 ==
  in : Inport  OutDataTypeStr=fixdt(0, 64, 0)  PortDimensions=1  SampleTime=1e-08
  Bit Shift2 : hdlsllib/Logic and Bit Operations/Bit Shift  mode=Shift Right Logical  N=double(1)
  Bit Slice2 : hdlsllib/Logic and Bit Operations/Bit Slice  lidx=double(0)  ridx=double(0)
  Data Type Conversion2 : DataTypeConversion  OutDataTypeStr=boolean  RndMeth=Nearest  SampleTime=1e-08  SaturateOnIntegerOverflow=off
  Switch2 : Switch  Criteria=u2 > Threshold  Threshold=double(0)  OutDataTypeStr=fixdt(0, 64, 0)  SampleTime=1e-08  SaturateOnIntegerOverflow=off  InputSameDT=off
  out : Outport  SampleTime=1e-08
  wires:
  in/1 -> Switch2/1, Bit Slice2/1, Bit Shift2/1
  Bit Shift2/1 -> Switch2/3
  Bit Slice2/1 -> Data Type Conversion2/1
  Data Type Conversion2/1 -> Switch2/2
  Switch2/1 -> out/1

== system gm_UZ_EnDat/UZ_ENDAT/ManualSerialize/padder/nibblepadding17/padding1 ==
  in : Inport  OutDataTypeStr=fixdt(0, 64, 0)  PortDimensions=1  SampleTime=1e-08
  Bit Shift2 : hdlsllib/Logic and Bit Operations/Bit Shift  mode=Shift Right Logical  N=double(1)
  Bit Slice2 : hdlsllib/Logic and Bit Operations/Bit Slice  lidx=double(0)  ridx=double(0)
  Data Type Conversion2 : DataTypeConversion  OutDataTypeStr=boolean  RndMeth=Nearest  SampleTime=1e-08  SaturateOnIntegerOverflow=off
  Switch2 : Switch  Criteria=u2 > Threshold  Threshold=double(0)  OutDataTypeStr=fixdt(0, 64, 0)  SampleTime=1e-08  SaturateOnIntegerOverflow=off  InputSameDT=off
  out : Outport  SampleTime=1e-08
  wires:
  Switch2/1 -> out/1
  Data Type Conversion2/1 -> Switch2/2
  Bit Slice2/1 -> Data Type Conversion2/1
  Bit Shift2/1 -> Switch2/3
  in/1 -> Bit Shift2/1, Bit Slice2/1, Switch2/1

== system gm_UZ_EnDat/UZ_ENDAT/ManualSerialize/padder/nibblepadding17/padding2 ==
  in : Inport  OutDataTypeStr=fixdt(0, 64, 0)  PortDimensions=1  SampleTime=1e-08
  Bit Shift2 : hdlsllib/Logic and Bit Operations/Bit Shift  mode=Shift Right Logical  N=double(1)
  Bit Slice2 : hdlsllib/Logic and Bit Operations/Bit Slice  lidx=double(0)  ridx=double(0)
  Data Type Conversion2 : DataTypeConversion  OutDataTypeStr=boolean  RndMeth=Nearest  SampleTime=1e-08  SaturateOnIntegerOverflow=off
  Switch2 : Switch  Criteria=u2 > Threshold  Threshold=double(0)  OutDataTypeStr=fixdt(0, 64, 0)  SampleTime=1e-08  SaturateOnIntegerOverflow=off  InputSameDT=off
  out : Outport  SampleTime=1e-08
  wires:
  in/1 -> Switch2/1, Bit Slice2/1, Bit Shift2/1
  Bit Shift2/1 -> Switch2/3
  Bit Slice2/1 -> Data Type Conversion2/1
  Data Type Conversion2/1 -> Switch2/2
  Switch2/1 -> out/1

== system gm_UZ_EnDat/UZ_ENDAT/ManualSerialize/padder/nibblepadding17/padding3 ==
  in : Inport  OutDataTypeStr=fixdt(0, 64, 0)  PortDimensions=1  SampleTime=1e-08
  Bit Shift2 : hdlsllib/Logic and Bit Operations/Bit Shift  mode=Shift Right Logical  N=double(1)
  Bit Slice2 : hdlsllib/Logic and Bit Operations/Bit Slice  lidx=double(0)  ridx=double(0)
  Data Type Conversion2 : DataTypeConversion  OutDataTypeStr=boolean  RndMeth=Nearest  SampleTime=1e-08  SaturateOnIntegerOverflow=off
  Switch2 : Switch  Criteria=u2 > Threshold  Threshold=double(0)  OutDataTypeStr=fixdt(0, 64, 0)  SampleTime=1e-08  SaturateOnIntegerOverflow=off  InputSameDT=off
  out : Outport  SampleTime=1e-08
  wires:
  in/1 -> Switch2/1, Bit Slice2/1, Bit Shift2/1
  Bit Shift2/1 -> Switch2/3
  Bit Slice2/1 -> Data Type Conversion2/1
  Data Type Conversion2/1 -> Switch2/2
  Switch2/1 -> out/1

== system gm_UZ_EnDat/UZ_ENDAT/ManualSerialize/padder/nibblepadding18/padding1 ==
  in : Inport  OutDataTypeStr=fixdt(0, 64, 0)  PortDimensions=1  SampleTime=1e-08
  Bit Shift2 : hdlsllib/Logic and Bit Operations/Bit Shift  mode=Shift Right Logical  N=double(1)
  Bit Slice2 : hdlsllib/Logic and Bit Operations/Bit Slice  lidx=double(0)  ridx=double(0)
  Data Type Conversion2 : DataTypeConversion  OutDataTypeStr=boolean  RndMeth=Nearest  SampleTime=1e-08  SaturateOnIntegerOverflow=off
  Switch2 : Switch  Criteria=u2 > Threshold  Threshold=double(0)  OutDataTypeStr=fixdt(0, 64, 0)  SampleTime=1e-08  SaturateOnIntegerOverflow=off  InputSameDT=off
  out : Outport  SampleTime=1e-08
  wires:
  Switch2/1 -> out/1
  Data Type Conversion2/1 -> Switch2/2
  Bit Slice2/1 -> Data Type Conversion2/1
  Bit Shift2/1 -> Switch2/3
  in/1 -> Bit Shift2/1, Bit Slice2/1, Switch2/1

== system gm_UZ_EnDat/UZ_ENDAT/ManualSerialize/padder/nibblepadding18/padding2 ==
  in : Inport  OutDataTypeStr=fixdt(0, 64, 0)  PortDimensions=1  SampleTime=1e-08
  Bit Shift2 : hdlsllib/Logic and Bit Operations/Bit Shift  mode=Shift Right Logical  N=double(1)
  Bit Slice2 : hdlsllib/Logic and Bit Operations/Bit Slice  lidx=double(0)  ridx=double(0)
  Data Type Conversion2 : DataTypeConversion  OutDataTypeStr=boolean  RndMeth=Nearest  SampleTime=1e-08  SaturateOnIntegerOverflow=off
  Switch2 : Switch  Criteria=u2 > Threshold  Threshold=double(0)  OutDataTypeStr=fixdt(0, 64, 0)  SampleTime=1e-08  SaturateOnIntegerOverflow=off  InputSameDT=off
  out : Outport  SampleTime=1e-08
  wires:
  in/1 -> Switch2/1, Bit Slice2/1, Bit Shift2/1
  Bit Shift2/1 -> Switch2/3
  Bit Slice2/1 -> Data Type Conversion2/1
  Data Type Conversion2/1 -> Switch2/2
  Switch2/1 -> out/1

== system gm_UZ_EnDat/UZ_ENDAT/ManualSerialize/padder/nibblepadding18/padding3 ==
  in : Inport  OutDataTypeStr=fixdt(0, 64, 0)  PortDimensions=1  SampleTime=1e-08
  Bit Shift2 : hdlsllib/Logic and Bit Operations/Bit Shift  mode=Shift Right Logical  N=double(1)
  Bit Slice2 : hdlsllib/Logic and Bit Operations/Bit Slice  lidx=double(0)  ridx=double(0)
  Data Type Conversion2 : DataTypeConversion  OutDataTypeStr=boolean  RndMeth=Nearest  SampleTime=1e-08  SaturateOnIntegerOverflow=off
  Switch2 : Switch  Criteria=u2 > Threshold  Threshold=double(0)  OutDataTypeStr=fixdt(0, 64, 0)  SampleTime=1e-08  SaturateOnIntegerOverflow=off  InputSameDT=off
  out : Outport  SampleTime=1e-08
  wires:
  in/1 -> Switch2/1, Bit Slice2/1, Bit Shift2/1
  Bit Shift2/1 -> Switch2/3
  Bit Slice2/1 -> Data Type Conversion2/1
  Data Type Conversion2/1 -> Switch2/2
  Switch2/1 -> out/1

== system gm_UZ_EnDat/UZ_ENDAT/ManualSerialize/padder/nibblepadding19/padding1 ==
  in : Inport  OutDataTypeStr=fixdt(0, 64, 0)  PortDimensions=1  SampleTime=1e-08
  Bit Shift2 : hdlsllib/Logic and Bit Operations/Bit Shift  mode=Shift Right Logical  N=double(1)
  Bit Slice2 : hdlsllib/Logic and Bit Operations/Bit Slice  lidx=double(0)  ridx=double(0)
  Data Type Conversion2 : DataTypeConversion  OutDataTypeStr=boolean  RndMeth=Nearest  SampleTime=1e-08  SaturateOnIntegerOverflow=off
  Switch2 : Switch  Criteria=u2 > Threshold  Threshold=double(0)  OutDataTypeStr=fixdt(0, 64, 0)  SampleTime=1e-08  SaturateOnIntegerOverflow=off  InputSameDT=off
  out : Outport  SampleTime=1e-08
  wires:
  Switch2/1 -> out/1
  Data Type Conversion2/1 -> Switch2/2
  Bit Slice2/1 -> Data Type Conversion2/1
  Bit Shift2/1 -> Switch2/3
  in/1 -> Bit Shift2/1, Bit Slice2/1, Switch2/1

== system gm_UZ_EnDat/UZ_ENDAT/ManualSerialize/padder/nibblepadding19/padding2 ==
  in : Inport  OutDataTypeStr=fixdt(0, 64, 0)  PortDimensions=1  SampleTime=1e-08
  Bit Shift2 : hdlsllib/Logic and Bit Operations/Bit Shift  mode=Shift Right Logical  N=double(1)
  Bit Slice2 : hdlsllib/Logic and Bit Operations/Bit Slice  lidx=double(0)  ridx=double(0)
  Data Type Conversion2 : DataTypeConversion  OutDataTypeStr=boolean  RndMeth=Nearest  SampleTime=1e-08  SaturateOnIntegerOverflow=off
  Switch2 : Switch  Criteria=u2 > Threshold  Threshold=double(0)  OutDataTypeStr=fixdt(0, 64, 0)  SampleTime=1e-08  SaturateOnIntegerOverflow=off  InputSameDT=off
  out : Outport  SampleTime=1e-08
  wires:
  in/1 -> Switch2/1, Bit Slice2/1, Bit Shift2/1
  Bit Shift2/1 -> Switch2/3
  Bit Slice2/1 -> Data Type Conversion2/1
  Data Type Conversion2/1 -> Switch2/2
  Switch2/1 -> out/1

== system gm_UZ_EnDat/UZ_ENDAT/ManualSerialize/padder/nibblepadding19/padding3 ==
  in : Inport  OutDataTypeStr=fixdt(0, 64, 0)  PortDimensions=1  SampleTime=1e-08
  Bit Shift2 : hdlsllib/Logic and Bit Operations/Bit Shift  mode=Shift Right Logical  N=double(1)
  Bit Slice2 : hdlsllib/Logic and Bit Operations/Bit Slice  lidx=double(0)  ridx=double(0)
  Data Type Conversion2 : DataTypeConversion  OutDataTypeStr=boolean  RndMeth=Nearest  SampleTime=1e-08  SaturateOnIntegerOverflow=off
  Switch2 : Switch  Criteria=u2 > Threshold  Threshold=double(0)  OutDataTypeStr=fixdt(0, 64, 0)  SampleTime=1e-08  SaturateOnIntegerOverflow=off  InputSameDT=off
  out : Outport  SampleTime=1e-08
  wires:
  in/1 -> Switch2/1, Bit Slice2/1, Bit Shift2/1
  Bit Shift2/1 -> Switch2/3
  Bit Slice2/1 -> Data Type Conversion2/1
  Data Type Conversion2/1 -> Switch2/2
  Switch2/1 -> out/1

== system gm_UZ_EnDat/UZ_ENDAT/ManualSerialize/padder/nibblepadding2/padding1 ==
  in : Inport  OutDataTypeStr=fixdt(0, 64, 0)  PortDimensions=1  SampleTime=1e-08
  Bit Shift2 : hdlsllib/Logic and Bit Operations/Bit Shift  mode=Shift Right Logical  N=double(1)
  Bit Slice2 : hdlsllib/Logic and Bit Operations/Bit Slice  lidx=double(0)  ridx=double(0)
  Data Type Conversion2 : DataTypeConversion  OutDataTypeStr=boolean  RndMeth=Nearest  SampleTime=1e-08  SaturateOnIntegerOverflow=off
  Switch2 : Switch  Criteria=u2 > Threshold  Threshold=double(0)  OutDataTypeStr=fixdt(0, 64, 0)  SampleTime=1e-08  SaturateOnIntegerOverflow=off  InputSameDT=off
  out : Outport  SampleTime=1e-08
  wires:
  Switch2/1 -> out/1
  Data Type Conversion2/1 -> Switch2/2
  Bit Slice2/1 -> Data Type Conversion2/1
  Bit Shift2/1 -> Switch2/3
  in/1 -> Bit Shift2/1, Bit Slice2/1, Switch2/1

== system gm_UZ_EnDat/UZ_ENDAT/ManualSerialize/padder/nibblepadding2/padding2 ==
  in : Inport  OutDataTypeStr=fixdt(0, 64, 0)  PortDimensions=1  SampleTime=1e-08
  Bit Shift2 : hdlsllib/Logic and Bit Operations/Bit Shift  mode=Shift Right Logical  N=double(1)
  Bit Slice2 : hdlsllib/Logic and Bit Operations/Bit Slice  lidx=double(0)  ridx=double(0)
  Data Type Conversion2 : DataTypeConversion  OutDataTypeStr=boolean  RndMeth=Nearest  SampleTime=1e-08  SaturateOnIntegerOverflow=off
  Switch2 : Switch  Criteria=u2 > Threshold  Threshold=double(0)  OutDataTypeStr=fixdt(0, 64, 0)  SampleTime=1e-08  SaturateOnIntegerOverflow=off  InputSameDT=off
  out : Outport  SampleTime=1e-08
  wires:
  in/1 -> Switch2/1, Bit Slice2/1, Bit Shift2/1
  Bit Shift2/1 -> Switch2/3
  Bit Slice2/1 -> Data Type Conversion2/1
  Data Type Conversion2/1 -> Switch2/2
  Switch2/1 -> out/1

== system gm_UZ_EnDat/UZ_ENDAT/ManualSerialize/padder/nibblepadding2/padding3 ==
  in : Inport  OutDataTypeStr=fixdt(0, 64, 0)  PortDimensions=1  SampleTime=1e-08
  Bit Shift2 : hdlsllib/Logic and Bit Operations/Bit Shift  mode=Shift Right Logical  N=double(1)
  Bit Slice2 : hdlsllib/Logic and Bit Operations/Bit Slice  lidx=double(0)  ridx=double(0)
  Data Type Conversion2 : DataTypeConversion  OutDataTypeStr=boolean  RndMeth=Nearest  SampleTime=1e-08  SaturateOnIntegerOverflow=off
  Switch2 : Switch  Criteria=u2 > Threshold  Threshold=double(0)  OutDataTypeStr=fixdt(0, 64, 0)  SampleTime=1e-08  SaturateOnIntegerOverflow=off  InputSameDT=off
  out : Outport  SampleTime=1e-08
  wires:
  in/1 -> Switch2/1, Bit Slice2/1, Bit Shift2/1
  Bit Shift2/1 -> Switch2/3
  Bit Slice2/1 -> Data Type Conversion2/1
  Data Type Conversion2/1 -> Switch2/2
  Switch2/1 -> out/1

== system gm_UZ_EnDat/UZ_ENDAT/ManualSerialize/padder/nibblepadding20/padding1 ==
  in : Inport  OutDataTypeStr=fixdt(0, 64, 0)  PortDimensions=1  SampleTime=1e-08
  Bit Shift2 : hdlsllib/Logic and Bit Operations/Bit Shift  mode=Shift Right Logical  N=double(1)
  Bit Slice2 : hdlsllib/Logic and Bit Operations/Bit Slice  lidx=double(0)  ridx=double(0)
  Data Type Conversion2 : DataTypeConversion  OutDataTypeStr=boolean  RndMeth=Nearest  SampleTime=1e-08  SaturateOnIntegerOverflow=off
  Switch2 : Switch  Criteria=u2 > Threshold  Threshold=double(0)  OutDataTypeStr=fixdt(0, 64, 0)  SampleTime=1e-08  SaturateOnIntegerOverflow=off  InputSameDT=off
  out : Outport  SampleTime=1e-08
  wires:
  Switch2/1 -> out/1
  Data Type Conversion2/1 -> Switch2/2
  Bit Slice2/1 -> Data Type Conversion2/1
  Bit Shift2/1 -> Switch2/3
  in/1 -> Bit Shift2/1, Bit Slice2/1, Switch2/1

== system gm_UZ_EnDat/UZ_ENDAT/ManualSerialize/padder/nibblepadding20/padding2 ==
  in : Inport  OutDataTypeStr=fixdt(0, 64, 0)  PortDimensions=1  SampleTime=1e-08
  Bit Shift2 : hdlsllib/Logic and Bit Operations/Bit Shift  mode=Shift Right Logical  N=double(1)
  Bit Slice2 : hdlsllib/Logic and Bit Operations/Bit Slice  lidx=double(0)  ridx=double(0)
  Data Type Conversion2 : DataTypeConversion  OutDataTypeStr=boolean  RndMeth=Nearest  SampleTime=1e-08  SaturateOnIntegerOverflow=off
  Switch2 : Switch  Criteria=u2 > Threshold  Threshold=double(0)  OutDataTypeStr=fixdt(0, 64, 0)  SampleTime=1e-08  SaturateOnIntegerOverflow=off  InputSameDT=off
  out : Outport  SampleTime=1e-08
  wires:
  in/1 -> Switch2/1, Bit Slice2/1, Bit Shift2/1
  Bit Shift2/1 -> Switch2/3
  Bit Slice2/1 -> Data Type Conversion2/1
  Data Type Conversion2/1 -> Switch2/2
  Switch2/1 -> out/1

== system gm_UZ_EnDat/UZ_ENDAT/ManualSerialize/padder/nibblepadding20/padding3 ==
  in : Inport  OutDataTypeStr=fixdt(0, 64, 0)  PortDimensions=1  SampleTime=1e-08
  Bit Shift2 : hdlsllib/Logic and Bit Operations/Bit Shift  mode=Shift Right Logical  N=double(1)
  Bit Slice2 : hdlsllib/Logic and Bit Operations/Bit Slice  lidx=double(0)  ridx=double(0)
  Data Type Conversion2 : DataTypeConversion  OutDataTypeStr=boolean  RndMeth=Nearest  SampleTime=1e-08  SaturateOnIntegerOverflow=off
  Switch2 : Switch  Criteria=u2 > Threshold  Threshold=double(0)  OutDataTypeStr=fixdt(0, 64, 0)  SampleTime=1e-08  SaturateOnIntegerOverflow=off  InputSameDT=off
  out : Outport  SampleTime=1e-08
  wires:
  in/1 -> Switch2/1, Bit Slice2/1, Bit Shift2/1
  Bit Shift2/1 -> Switch2/3
  Bit Slice2/1 -> Data Type Conversion2/1
  Data Type Conversion2/1 -> Switch2/2
  Switch2/1 -> out/1

== system gm_UZ_EnDat/UZ_ENDAT/ManualSerialize/padder/nibblepadding21/padding1 ==
  in : Inport  OutDataTypeStr=fixdt(0, 64, 0)  PortDimensions=1  SampleTime=1e-08
  Bit Shift2 : hdlsllib/Logic and Bit Operations/Bit Shift  mode=Shift Right Logical  N=double(1)
  Bit Slice2 : hdlsllib/Logic and Bit Operations/Bit Slice  lidx=double(0)  ridx=double(0)
  Data Type Conversion2 : DataTypeConversion  OutDataTypeStr=boolean  RndMeth=Nearest  SampleTime=1e-08  SaturateOnIntegerOverflow=off
  Switch2 : Switch  Criteria=u2 > Threshold  Threshold=double(0)  OutDataTypeStr=fixdt(0, 64, 0)  SampleTime=1e-08  SaturateOnIntegerOverflow=off  InputSameDT=off
  out : Outport  SampleTime=1e-08
  wires:
  Switch2/1 -> out/1
  Data Type Conversion2/1 -> Switch2/2
  Bit Slice2/1 -> Data Type Conversion2/1
  Bit Shift2/1 -> Switch2/3
  in/1 -> Bit Shift2/1, Bit Slice2/1, Switch2/1

== system gm_UZ_EnDat/UZ_ENDAT/ManualSerialize/padder/nibblepadding21/padding2 ==
  in : Inport  OutDataTypeStr=fixdt(0, 64, 0)  PortDimensions=1  SampleTime=1e-08
  Bit Shift2 : hdlsllib/Logic and Bit Operations/Bit Shift  mode=Shift Right Logical  N=double(1)
  Bit Slice2 : hdlsllib/Logic and Bit Operations/Bit Slice  lidx=double(0)  ridx=double(0)
  Data Type Conversion2 : DataTypeConversion  OutDataTypeStr=boolean  RndMeth=Nearest  SampleTime=1e-08  SaturateOnIntegerOverflow=off
  Switch2 : Switch  Criteria=u2 > Threshold  Threshold=double(0)  OutDataTypeStr=fixdt(0, 64, 0)  SampleTime=1e-08  SaturateOnIntegerOverflow=off  InputSameDT=off
  out : Outport  SampleTime=1e-08
  wires:
  in/1 -> Switch2/1, Bit Slice2/1, Bit Shift2/1
  Bit Shift2/1 -> Switch2/3
  Bit Slice2/1 -> Data Type Conversion2/1
  Data Type Conversion2/1 -> Switch2/2
  Switch2/1 -> out/1

== system gm_UZ_EnDat/UZ_ENDAT/ManualSerialize/padder/nibblepadding21/padding3 ==
  in : Inport  OutDataTypeStr=fixdt(0, 64, 0)  PortDimensions=1  SampleTime=1e-08
  Bit Shift2 : hdlsllib/Logic and Bit Operations/Bit Shift  mode=Shift Right Logical  N=double(1)
  Bit Slice2 : hdlsllib/Logic and Bit Operations/Bit Slice  lidx=double(0)  ridx=double(0)
  Data Type Conversion2 : DataTypeConversion  OutDataTypeStr=boolean  RndMeth=Nearest  SampleTime=1e-08  SaturateOnIntegerOverflow=off
  Switch2 : Switch  Criteria=u2 > Threshold  Threshold=double(0)  OutDataTypeStr=fixdt(0, 64, 0)  SampleTime=1e-08  SaturateOnIntegerOverflow=off  InputSameDT=off
  out : Outport  SampleTime=1e-08
  wires:
  in/1 -> Switch2/1, Bit Slice2/1, Bit Shift2/1
  Bit Shift2/1 -> Switch2/3
  Bit Slice2/1 -> Data Type Conversion2/1
  Data Type Conversion2/1 -> Switch2/2
  Switch2/1 -> out/1
